simulink model "Stability_Study_QUATERNION_moments"  (R2019a)
settings: Solver=VariableStepAuto  StartTime=0.0  StopTime=100.0  RelTol=1e-3
undefined symbols (not defined in the file): psi, psi_dot, w, x, x0_dot, x0_dotdot, x_dot
libraries: sharedutil x2, aerolibnav x2, shared6dof x1
settings Model: Creator=thibault  LastModifiedBy=thibault
settings DataIOCC: ReturnWorkspaceOutputs=off
settings DebuggingCC: PregeneratedLibrarySubsystemCodeDiagnostic=none  ArithmeticOperatorsInVariantConditions=warning
settings SFSimCC: SimUseLocalCustomCode=off
settings RTWCC: RTWUseLocalCustomCode=off

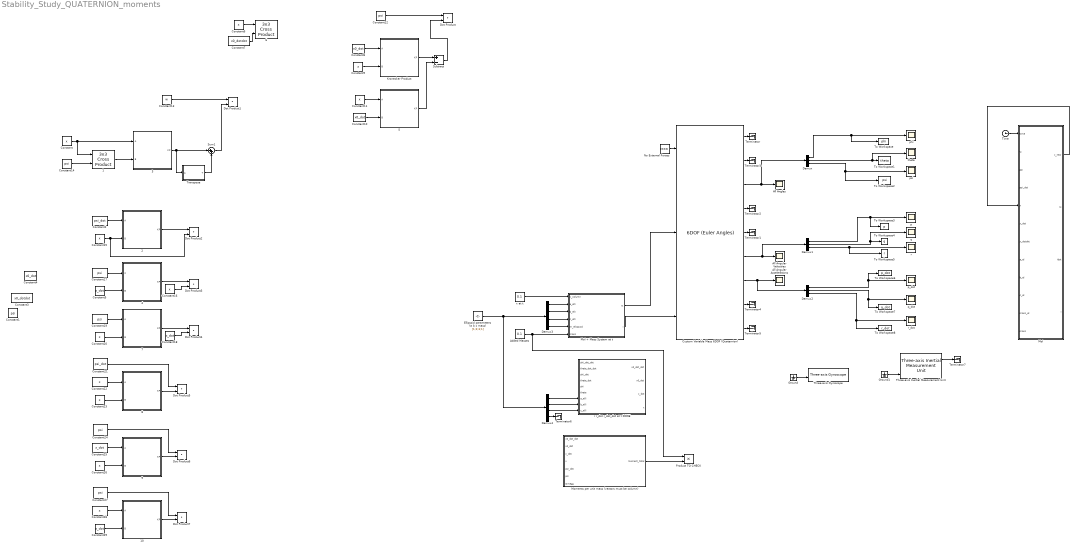
== system Stability_Study_QUATERNION_moments ==
  1 : sharedutil/3x3 Cross Product  aMode=aMode
      settings: SourceProductBaseCode=AE
  10 : MATLAB Function  TreatAsAtomicUnit=on
  2 : MATLAB Function  TreatAsAtomicUnit=on
  3 : MATLAB Function  TreatAsAtomicUnit=on
  4 : MATLAB Function  TreatAsAtomicUnit=on
  5 : MATLAB Function  TreatAsAtomicUnit=on
  6 : sharedutil/3x3 Cross Product  aMode=aMode
      settings: SourceProductBaseCode=AE
  7 : MATLAB Function  TreatAsAtomicUnit=on
  8 : MATLAB Function  TreatAsAtomicUnit=on
  9 : MATLAB Function  TreatAsAtomicUnit=on
  Added Masses : Constant  Value=0.1
  All Angles : Scope
  All Angular Accelerations : Scope
  All Angular Velocities : Scope
  Constant{,6,9,11,15..16,20,22..23,26,28} (11 alike) : Constant  Value=x
  Constant{1,12,14,17,19,24,27} (7 alike) : Constant  Value=psi
  Constant10 : Constant  Value=x0_dot
  Constant13 : Constant  Value=w
  Constant{5,18,25,29} (4 alike) : Constant  Value=x_dot
  Constant2 : Constant  Value=psi_dot
  Constant21 : Constant  Value=psi_dot
  Constant3 : Constant  Value=x0_dotdot
  Constant4 : Constant  Value=x0_dot
  Constant7 : Constant  Value=x0_dotdot
  Constant8 : Constant  Value=x0_dot
  Custom Variable Mass 6DOF (Quaternion) : shared6dof/6DOF (Euler Angles)  units=Metric (MKS)  mtype=Custom Variable  rep=Quaternion  xme_0=[0 0 0]  Vm_0=[0 0 0]  eul_0=[0 0 0]  pm_0=[0 0 1]  mass_0=1.0  mass_e=0.5  mass_f=2.0  inertia=eye(3)  inertia_e=eye(3)  inertia_f=2*eye(3)  k_quat=1.0  vre_flag=off  abi_flag=on  aMode=0  xme_statename=''  Vm_statename=''  eul_statename=''  quat_statename=''  pm_statename=''  mass_statename=''
      settings: SourceProductBaseCode=AE
  Demux : Demux  Outputs=3
  Demux1 : Demux  Outputs=3
  Demux2 : Demux  Outputs=3
  Demux3 : Demux
  Demux4 : Demux
  Dot Product{,1..7} (8 alike) : DotProduct  InputSameDT=on  OutDataTypeStr=Inherit: Inherit via internal rule
  Ellipsoid parameters (a b c mass) : Constant  Value=[1;2;3;1]  VectorParams1D=off
  Ground : Ground
  Ground1 : Ground
  Kronecker Product : MATLAB Function  TreatAsAtomicUnit=on
  MoI : MATLAB Function  TreatAsAtomicUnit=on
  MoI + Mass System at t : MATLAB Function  TreatAsAtomicUnit=on
  Moments per unit mass (vectors must be column) : MATLAB Function  TreatAsAtomicUnit=on
  No External Forces : Constant  Value=[0;0;0]
  Product TO CHECK : Product
  Subtract : Sum  Inputs=+-
  Sum1 : Sum  Inputs=|++
  Terminator{,1..7} (8 alike) : Terminator
  Three-axis Gyroscope : aerolibnav/Three-axis Gyroscope  dtype_g=on  w_g=190  z_g=0.707  g_sf_cc=[1 0 0; 0 1 0; 0 0 1]  g_bias=[0 0 0]  g_sen=[0 0 0]  g_Ts=0  g_rand=on  g_seeds=[23093 23094 23095]  g_pow=[0.0001 0.0001 0.0001]  g_sat="[-inf  -inf  -inf  inf inf inf]"
      settings: SourceProductName=Aerospace Blockset  SourceProductBaseCode=AE
  Three-axis Inertial Measurement Unit : aerolibnav/Three-axis Inertial Measurement Unit  units=Metric (MKS)  imu=[0 0 0]  i_Ts=0  dtype_a=on  w_a=190  z_a=0.707  a_sf_cc=[1 0 0; 0 1 0; 0 0 1]  a_bias=[0 0 0]  a_sat="[-inf  -inf  -inf  inf inf inf]"  dtype_g=on  w_g=190  z_g=0.707  g_sf_cc=[1 0 0; 0 1 0; 0 0 1]  g_bias=[0 0 0]  g_sens=[0 0 0]  g_sat="[-inf  -inf  -inf  inf inf inf]"  i_rand=on  i_seeds=[23093 23094 23095 23096 23097 23098]  i_pow=[0.001 0.001 0.001 0.0001 0.0001 0.0001]
  Time : Clock
      settings: Decimation=1000
  To Workspace : ToWorkspace  VariableName=phi  SaveFormat=Timeseries  SampleTime=-1
  To Workspace1 : ToWorkspace  VariableName=theta  SaveFormat=Timeseries  SampleTime=-1
  To Workspace2 : ToWorkspace  VariableName=psi  SaveFormat=Timeseries  SampleTime=-1
  To Workspace3 : ToWorkspace  VariableName=p  SaveFormat=Timeseries  SampleTime=-1
  To Workspace4 : ToWorkspace  VariableName=q  SaveFormat=Timeseries  SampleTime=-1
  To Workspace5 : ToWorkspace  VariableName=r  SaveFormat=Timeseries  SampleTime=-1
  To Workspace6 : ToWorkspace  VariableName=p_dot  SaveFormat=Timeseries  SampleTime=-1
  To Workspace7 : ToWorkspace  VariableName=q_dot  SaveFormat=Timeseries  SampleTime=-1
  To Workspace8 : ToWorkspace  VariableName=r_dot  SaveFormat=Timeseries  SampleTime=-1
  Transpose : MATLAB Function  TreatAsAtomicUnit=on
  p : Scope
  p_dot : Scope
  phi : Scope
  psi : Scope
  q : Scope
  q_dot : Scope
  r : Scope
  r r_dot r_dot_dot at t DONE : MATLAB Function  TreatAsAtomicUnit=on
  r_dot : Scope
  theta : Scope
  x at t : Constant  Value=0.1
  wires:
  No External Forces/1 -> Custom Variable Mass 6DOF (Quaternion)/1
  Custom Variable Mass 6DOF (Quaternion)/1 -> Terminator/1
  Custom Variable Mass 6DOF (Quaternion)/2 -> Terminator3/1
  Custom Variable Mass 6DOF (Quaternion)/4 -> Terminator2/1
  Custom Variable Mass 6DOF (Quaternion)/5 -> Terminator1/1
  Custom Variable Mass 6DOF (Quaternion)/3 -> Demux/1, All Angles/1
  Demux/1 -> To Workspace/1, phi/1
  Demux/2 -> To Workspace1/1, theta/1
  Demux/3 -> To Workspace2/1, psi/1
  Custom Variable Mass 6DOF (Quaternion)/8 -> Terminator4/1
  Custom Variable Mass 6DOF (Quaternion)/9 -> Terminator5/1
  Custom Variable Mass 6DOF (Quaternion)/6 -> Demux1/1, All Angular Velocities/1
  Demux1/1 -> To Workspace3/1, p/1
  Demux1/2 -> q/1, To Workspace4/1
  Demux1/3 -> To Workspace5/1, r/1
  Demux2/1 -> To Workspace6/1, p_dot/1
  Demux2/2 -> To Workspace7/1, q_dot/1
  Demux2/3 -> To Workspace8/1, r_dot/1
  Custom Variable Mass 6DOF (Quaternion)/7 -> Demux2/1, All Angular Accelerations/1
  Ellipsoid parameters (a b c mass)/1 -> Demux4/1, Demux3/1
  Time/1 -> MoI/1(time)
  MoI/1(x_new) -> MoI/5(x)
  Constant7/1 -> 6/2
  Constant6/1 -> 6/1
  Constant8/1 -> Kronecker Product/1(A)
  Constant9/1 -> Kronecker Product/2(B)
  Constant11/1 -> 5/1(A)
  Constant10/1 -> 5/2(B)
  Constant12/1 -> Dot Product/1
  Kronecker Product/1(KP) -> Subtract/1
  5/1(KP) -> Subtract/2
  Subtract/1 -> Dot Product/2
  Constant13/1 -> Dot Product1/1
  Constant/1 -> 1/1, 3/1(A)
  Constant14/1 -> 1/2
  1/1 -> 3/2(B)
  3/1(KP) -> Transpose/1(A), Sum1/1
  Sum1/1 -> Dot Product1/2
  Transpose/1(T) -> Sum1/2
  Constant2/1 -> 2/1(A)
  Constant15/1 -> Dot Product2/2, 2/2(B)
  2/1(KP) -> Dot Product2/1
  4/1(KP) -> Dot Product3/1
  Constant17/1 -> 4/1(A)
  Constant5/1 -> 4/2(B)
  Constant16/1 -> Dot Product3/2
  Constant18/1 -> Dot Product4/2
  7/1(KP) -> Dot Product4/1
  Constant19/1 -> 7/1(A)
  Constant20/1 -> 7/2(B)
  Constant22/1 -> 8/1(A)
  Constant23/1 -> 8/2(B)
  8/1(KP) -> Dot Product5/2
  Constant21/1 -> Dot Product5/1
  Constant24/1 -> Dot Product6/1
  9/1(KP) -> Dot Product6/2
  Constant25/1 -> 9/1(A)
  Constant26/1 -> 9/2(B)
  Constant28/1 -> 10/1(A)
  10/1(KP) -> Dot Product7/2
  Constant27/1 -> Dot Product7/1
  Constant29/1 -> 10/2(B)
  MoI + Mass System at t/2(I) -> Custom Variable Mass 6DOF (Quaternion)/5
  x at t/1 -> MoI + Mass System at t/1(x_column)
  Demux3/4 -> MoI + Mass System at t/5(m_ellipsoid)
  Demux3/3 -> MoI + Mass System at t/4(c_elli)
  Demux3/2 -> MoI + Mass System at t/3(b_elli)
  Demux3/1 -> MoI + Mass System at t/2(a_elli)
  Added Masses/1 -> Product TO CHECK/1, MoI + Mass System at t/6(mass)
  MoI + Mass System at t/1(m) -> Custom Variable Mass 6DOF (Quaternion)/3
  Demux4/4 -> Terminator6/1
  Demux4/3 -> r r_dot r_dot_dot at t DONE/9(c_elli)
  Demux4/2 -> r r_dot r_dot_dot at t DONE/8(b_elli)
  Demux4/1 -> r r_dot r_dot_dot at t DONE/7(a_elli)
  Ground/1 -> Three-axis Gyroscope/2
  Ground1/1 -> Three-axis Inertial Measurement Unit/5
  Three-axis Inertial Measurement Unit/1 -> Terminator7/1
  Moments per unit mass (vectors must be column)/1(moment_total) -> Product TO CHECK/2

== matlab function Stability_Study_QUATERNION_moments/Kronecker Product ==
  data: KP output; A input; B input
function KP = Kronecker(A, B)
KP=kron(A,B);
end

== matlab function Stability_Study_QUATERNION_moments/5 ==
  data: KP output; A input; B input
function KP = Kronecker(A, B)
KP=kron(A,B);
end

== matlab function Stability_Study_QUATERNION_moments/MoI ==
  data: x_new output; M output; time input; w input; psi input; Idot output; psi_dot input; x input; x_dot input; x_dotdot input; I output; a_el input; b_el input; c_el input; mass_el input; mass input
function [x_new, M, Idot, I] = MoI(time, w, psi, psi_dot,x,x_dot,x_dotdot, a_el, b_el, c_el, mass_el, mass)
%x0!!!!!! TO ADD
tp=
dt=time-tp;
%Moment of inertia ellipsoid + mass DONE
%===============================================================================
a=a_el;
b=b_el;
c=c_el;
I=0.2*mass_el*[b^2+c^2 0 0;
               0 a^2+c^2 0;
               0 0 a^2+b^2]+mass*((x*x.')*eye(3)-kron(x,x.')); %assuming x column vector
%===========================================================================================

%Time differentiation of MoI
Idot=2*mass*((x_dot*x.')*eye(3)-kron(x_dot,x.'));

tp=time;

x_new=x_dot*dt+x;

M=cross(x,x_dot);
M=M-w*((cross(kron(x,x),psi)+(cross(kron(x,x),psi).')));
M=M+(kron(psi_dot,x)*x+kron(psi,x_dot)*x+kron(psi,x)*x_dot-psi_dot*kron(x,x)-psi*kron(x_dot,x)-psi*kron(x,x_dot));

M=M+cross(x,x_dotdot);
M=mass*M;
end

== matlab function Stability_Study_QUATERNION_moments/3 ==
  data: KP output; A input; B input
function KP = Kronecker(A, B) %dont forget to input A and B as column
KP=kron(A,B');
end

== matlab function Stability_Study_QUATERNION_moments/Transpose ==
  data: T output; A input
function T = Transpose(A) 
T=A';
end

== matlab function Stability_Study_QUATERNION_moments/2 ==
  data: KP output; A input; B input
function KP = Kronecker(A, B) %dont forget to input A and B as column
KP=kron(A,B');
end

== matlab function Stability_Study_QUATERNION_moments/4 ==
  data: KP output; A input; B input
function KP = Kronecker(A, B) %dont forget to input A and B as column
KP=kron(A,B');
end

== matlab function Stability_Study_QUATERNION_moments/7 ==
  data: KP output; A input; B input
function KP = Kronecker(A, B) %dont forget to input A and B as column
KP=kron(A,B');
end

== matlab function Stability_Study_QUATERNION_moments/8 ==
  data: KP output; A input; B input
function KP = Kronecker(A, B) %dont forget to input A and B as column
KP=kron(A,B');
end

== matlab function Stability_Study_QUATERNION_moments/9 ==
  data: KP output; A input; B input
function KP = Kronecker(A, B) %dont forget to input A and B as column
KP=kron(A,B');
end

== matlab function Stability_Study_QUATERNION_moments/10 ==
  data: KP output; A input; B input
function KP = Kronecker(A, B) %dont forget to input A and B as column
KP=kron(A,B');
end

== matlab function Stability_Study_QUATERNION_moments/MoI + Mass System at t ==
  data: m output; x_column input; a_elli input; b_elli input; c_elli input; m_ellipsoid input; I output; mass input
function [m, I] = MoI(x_column, a_elli, b_elli, c_elli, m_ellipsoid, mass)

m=mass+m_ellipsoid; %total mass

a=a_elli;
b=b_elli;
c=c_elli;

x=x_column;

I=0.2*m_ellipsoid*[b^2+c^2 0 0;
               0 a^2+c^2 0;
               0 0 a^2+b^2]+mass*(dot(x,x)*eye(3)-kron(x,x')); %assuming x column vector
end

== matlab function Stability_Study_QUATERNION_moments/r r_dot r_dot_dot at t DONE ==
  data: phi_dot_dot input; x0_dot_dot output; theta_dot_dot input; phi_dot input; theta_dot input; phi input; theta input; x0_dot output; x_dot output; a_elli input; b_elli input; c_elli input; x output
function [x0_dot_dot,x0_dot,x_dot,x] = radii(phi_dot_dot, theta_dot_dot, phi_dot, theta_dot, phi, theta, a_elli, b_elli, c_elli)

%ellipsoid parmeters
a2 = a_elli^2;
b2 = b_elli^2;
c2 = c_elli^2;

%angles and angular velocities
phidd = phi_dot_dot;
thetadd = theta_dot_dot;
phid = phi_dot;
thetad = theta_dot;

%trigonometric function calculated only once!!
cosp = cos(phi);
sinp = sin(phi);
cos2p = cos(2*phi);
sin2p = sin(2*phi);
cost = cos(theta);
sint = sin(theta);
cos2t = cos(2*theta);
sin2t = sin(2*theta);

%OK done base
base = (cosp^2)*(sint^2)/a2 + (sinp^2)*(sint^2)/b2 + cost^2/c2;

%OK prime done
prime = (cosp^2*sin2t*thetad - sin2p*phid*sint^2)/a2 + (sinp^2*sin2t*thetad + sin2p*phid*sint^2)/b2 - (sin2t*thetad)/c2;

%OK second done
prime_a_dot = (cosp^2*cos2t*2*thetad^2 + cosp^2*sin2t*thetadd - 2*sin2p*phid*sin2t*thetad - 2*cos2p*phid^2*sint^2 - sin2p*phidd*sint^2)/a2; %done
prime_b_dot = (sinp^2*2*cos2t*thetad^2 + sinp^2*sin2t*thetadd + 2*sin2p*phid*sin2t*thetad + 2*cos2p*phid^2*sint^2 + sin2p*phidd*sint^2)/b2; %done
prime_c_dot = -(2*cos2t*thetad^2 + sin2t*thetadd)/c2; %done

second = prime_a_dot + prime_b_dot + prime_c_dot;

r = sqrt(1/base); %done
r_dot = -0.5*r^3*prime; %done
r_dot_dot = 0.75*r^5*prime^2 - 0.5*r^3*second; %done

e_r = [cosp*sint;sinp*sint;cost]; %done
e_phi = [-sinp;cosp;0]; %done
e_theta = [cosp*cost;sinp*cost;-sint]; %done

x = r*e_r; %done
x_dot = r_dot*e_r + r*(phid*sint*e_phi + thetad*e_theta); %done
x0_dot = r_dot*e_r; %done
x0_dot_dot = r_dot_dot*e_r; %done
end

== matlab function Stability_Study_QUATERNION_moments/Moments per unit mass (vectors must be column) ==
  data: x0_dot_dot input; x0_dot input; x_dot input; x input; psi_dot input; psi input; Omega input; moment_total output
function moment_total = moments(x0_dot_dot,x0_dot, x_dot,x, psi_dot, psi, Omega)

%All vectors must be column vectors
%All moments are per unit mass the output must be multiplied by the mass

w=Omega;

momentJ=-2*(dot(x0_dot,x)*eye(3)-kron(x0_dot,x'))*w;
moment1=-(kron(x,x0_dot)-kron(x0_dot,x'))*psi;
moment2=-()*w
moment3=-cross(x,x0_dot_dot);
moment4=-();

moment_total = momentJ+moment1+moment2+moment3+moment4;
end
